simulink model "model"  (R2019b)
settings: Solver=VariableStepAuto  StartTime=0.0  StopTime=20.0  RelTol=1e-3
settings Model: Creator=Mustafa Sezer  LastModifiedBy=Mustafa Sezer

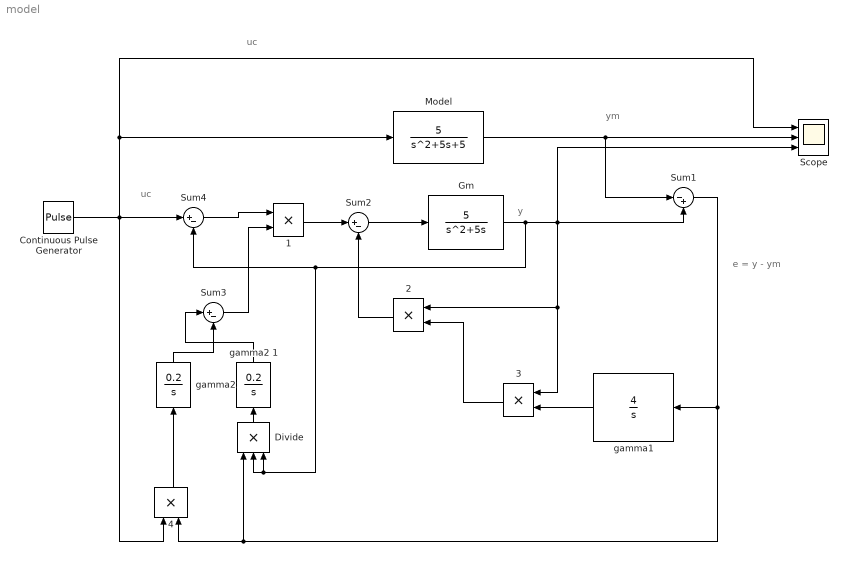
== system model ==
  note: e = y - ym
  note: uc
  note: uc
  note: ym
  note: y
   {1..4} (4 alike) : Product
  Continuous Pulse Generator : DiscretePulseGenerator  PulseType=Time based  Period=20  PulseWidth=50
  Divide : Product  Inputs=***
  "Gm  " : TransferFcn  Numerator=[5]  Denominator=[1 5 0]
  Model : TransferFcn  Numerator=[5]  Denominator=[1 5 5]
  Scope : Scope  NumInputPorts=3
  Sum1 : Sum  Inputs=|-+
  Sum2 : Sum  Inputs=|+-
  Sum3 : Sum  Inputs=|+-
  Sum4 : Sum  Inputs=|+-
  gamma1 : TransferFcn  Numerator=[4]  Denominator=[1 0]
  "gamma2 " : TransferFcn  Numerator=[0.2]  Denominator=[1 0]
  gamma2 1 : TransferFcn  Numerator=[0.2]  Denominator=[1 0]
  wires:
  " 3"/1 -> " 2"/2
  " 2"/1 -> Sum2/2
  Sum2/1 -> "Gm  "/1
  gamma1/1 -> " 3"/2
  " 1"/1 -> Sum2/1
  Model/1 -> Scope/2, Sum1/1
  "Gm  "/1 -> Divide/3, Divide/2, Sum4/2, " 2"/1, " 3"/1, Scope/3, Sum1/2
  Continuous Pulse Generator/1 -> " 4"/1, Sum4/1, Model/1, Scope/1
  Sum4/1 -> " 1"/1
  " 4"/1 -> "gamma2 "/1
  Sum1/1 -> Divide/1, " 4"/2, gamma1/1
  Divide/1 -> gamma2 1/1
  gamma2 1/1 -> Sum3/1
  "gamma2 "/1 -> Sum3/2
  Sum3/1 -> " 1"/2
